simulink subsystem "s_parameters"  (R2024b)
settings: Solver=VariableStepAuto  StartTime=0.0  StopTime=10.0  RelTol=1e-3
settings Model: Creator=marwa  LastModifiedBy=marwa

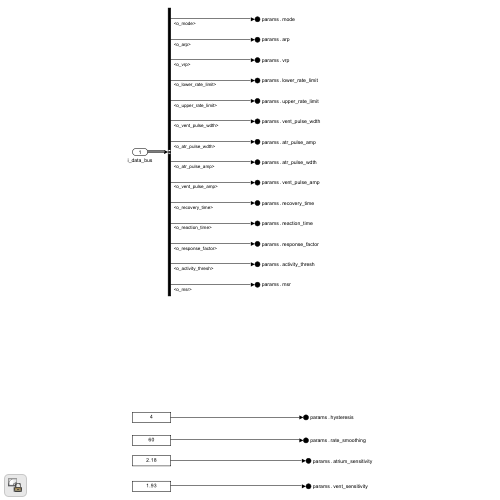
[thumbnail: Simulink's stored preview of the top-level diagram]
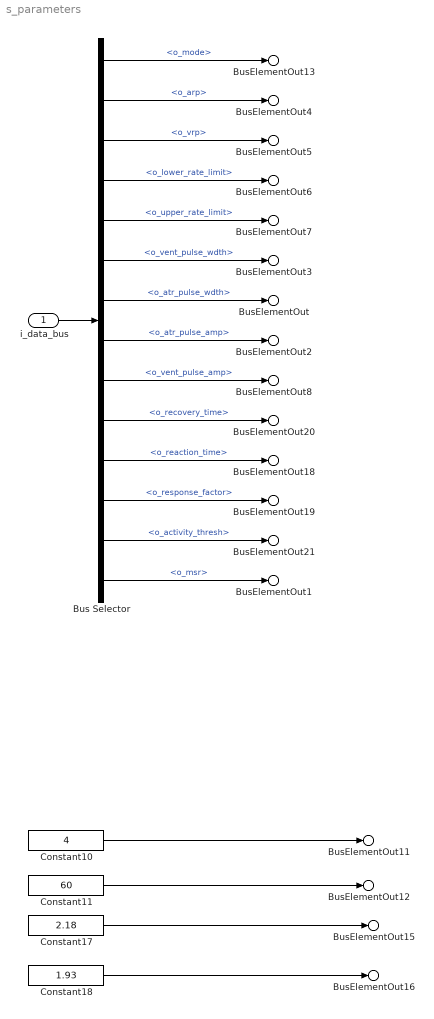
== system s_parameters ==
  i_data_bus : Inport
  Bus Selector : BusSelector  OutputSignals=o_mode,o_arp,o_vrp,o_lower_rate_limit,o_upper_rate_limit,o_vent_pulse_wdth,o_atr_pulse_wdth,o_atr_pulse_amp,o_vent_pulse_amp,o_recovery_time,o_reaction_time,o_response_factor,o_activity_thresh,o_msr
  Constant10 : Constant  Value=4
  Constant11 : Constant  Value=60
  Constant17 : Constant  Value=2.18
  Constant18 : Constant  Value=1.93
  BusElementOut11 : Outport  PortName=params  Element=hysteresis
  BusElementOut12 : Outport  PortName=params  Element=rate_smoothing
  BusElementOut13 : Outport  PortName=params  Element=mode
  BusElementOut15 : Outport  PortName=params  Element=atrium_sensitivity
  BusElementOut16 : Outport  PortName=params  Element=vent_sensitivity
  BusElementOut18 : Outport  PortName=params  Element=reaction_time
  BusElementOut19 : Outport  PortName=params  Element=response_factor
  BusElementOut20 : Outport  PortName=params  Element=recovery_time
  BusElementOut21 : Outport  PortName=params  Element=activity_thresh
  BusElementOut : Outport  PortName=params  Element=atr_pulse_amp
  BusElementOut2 : Outport  PortName=params  Element=atr_pulse_wdth
  BusElementOut3 : Outport  PortName=params  Element=vent_pulse_wdth
  BusElementOut4 : Outport  PortName=params  Element=arp
  BusElementOut5 : Outport  PortName=params  Element=vrp
  BusElementOut6 : Outport  PortName=params  Element=lower_rate_limit
  BusElementOut7 : Outport  PortName=params  Element=upper_rate_limit
  BusElementOut8 : Outport  PortName=params  Element=vent_pulse_amp
  BusElementOut1 : Outport  PortName=params  Element=msr
  wires:
  i_data_bus/1 -> Bus Selector/1
  Bus Selector/1 -> BusElementOut13/1  "<o_mode>"
  Bus Selector/2 -> BusElementOut4/1  "<o_arp>"
  Bus Selector/3 -> BusElementOut5/1  "<o_vrp>"
  Bus Selector/5 -> BusElementOut7/1  "<o_upper_rate_limit>"
  Bus Selector/6 -> BusElementOut3/1  "<o_vent_pulse_wdth>"
  Bus Selector/4 -> BusElementOut6/1  "<o_lower_rate_limit>"
  Bus Selector/7 -> BusElementOut/1  "<o_atr_pulse_wdth>"
  Bus Selector/8 -> BusElementOut2/1  "<o_atr_pulse_amp>"
  Bus Selector/9 -> BusElementOut8/1  "<o_vent_pulse_amp>"
  Bus Selector/10 -> BusElementOut20/1  "<o_recovery_time>"
  Bus Selector/11 -> BusElementOut18/1  "<o_reaction_time>"
  Bus Selector/12 -> BusElementOut19/1  "<o_response_factor>"
  Bus Selector/13 -> BusElementOut21/1  "<o_activity_thresh>"
  Constant11/1 -> BusElementOut12/1
  Constant10/1 -> BusElementOut11/1
  Constant17/1 -> BusElementOut15/1
  Constant18/1 -> BusElementOut16/1
  Bus Selector/14 -> BusElementOut1/1  "<o_msr>"
